simulink model "backstepping"  (R2018a)
settings: Solver=VariableStepAuto  StartTime=0.0  StopTime=500  RelTol=1e-3
values from neighbouring files (symbols this model uses):
  D = 0    [k_func.m]
libraries: simulink_extras x4, sharedutil x3, dspmtrx3 x3
settings Model: Creator=Renz  LastModifiedBy=Renz

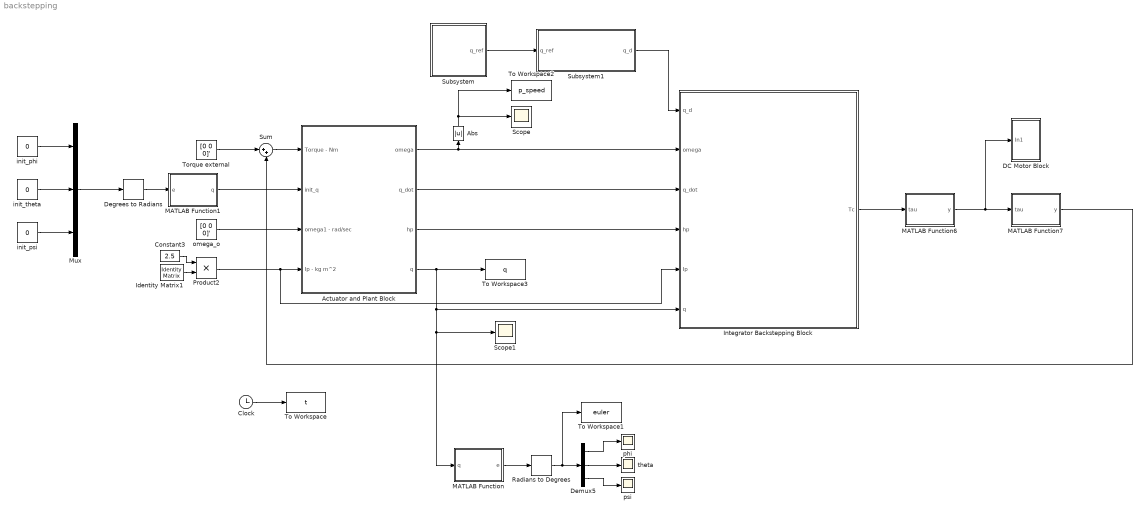
== system backstepping ==
  Abs : Abs
  Actuator and Plant Block : Subsystem
  Clock : Clock
  Constant3 : Constant  Value=2.5
  DC Motor Block : Subsystem
  Degrees to Radians : simulink_extras/Transformations/Degrees to Radians
  Demux5 : Demux  Outputs=3
  Identity Matrix1 : dspmtrx3/Identity Matrix  Inherit=off  N=3  Ts=1  dataType=double  isSigned=on  wordLen=16  udDataType=sfix(16)  fracBitsMode=Best precision  numFracBits=15  OutDataTypeStr=double  LastOutDataTypeStr=double
      settings: SourceProductName=DSP System Toolbox
  Integrator Backstepping Block : Subsystem
  MATLAB Function : MATLAB Function  TreatAsAtomicUnit=on
  MATLAB Function1 : MATLAB Function  TreatAsAtomicUnit=on
  MATLAB Function6 : MATLAB Function  TreatAsAtomicUnit=on
  MATLAB Function7 : MATLAB Function  TreatAsAtomicUnit=on
  Mux : Mux  Inputs=3
  Product2 : Product
  Radians to Degrees : simulink_extras/Transformations/Radians to Degrees
  Scope : Scope
  Scope1 : Scope
  Subsystem : Subsystem
  Subsystem1 : Subsystem
  Sum : Sum  Inputs=|++
  To Workspace : ToWorkspace  VariableName=t  SampleTime=-1
  To Workspace1 : ToWorkspace  VariableName=euler  SampleTime=-1
  To Workspace2 : ToWorkspace  VariableName=p_speed  SampleTime=-1
  To Workspace3 : ToWorkspace  VariableName=q  SampleTime=-1
  Torque external : Constant  Value=[0 0 0]'
  init_phi : Constant  Value=0
  init_psi : Constant  Value=0
  init_theta : Constant  Value=0
  "omega_o " : Constant  Value=[0 0 0]'
  phi : Scope
  psi : Scope
  theta : Scope
  wires:
  Identity Matrix1/1 -> Product2/2
  MATLAB Function1/1(q) -> Actuator and Plant Block/2(init_q)
  init_psi/1 -> Mux/3
  "omega_o "/1 -> Actuator and Plant Block/3(omega1 - rad/sec)
  Sum/1 -> Actuator and Plant Block/1(Torque - Nm)
  init_theta/1 -> Mux/2
  Demux5/3 -> psi/1
  Product2/1 -> Integrator Backstepping Block/5(Ip), Actuator and Plant Block/4(Ip - kg m^2)
  Demux5/1 -> phi/1
  Constant3/1 -> Product2/1
  Clock/1 -> To Workspace/1
  Subsystem/1(q_ref) -> Subsystem1/1(q_ref)
  Actuator and Plant Block/4(q) -> MATLAB Function/1(q), Scope1/1, Integrator Backstepping Block/6(q), To Workspace3/1
  Radians to Degrees/1 -> To Workspace1/1, Demux5/1
  Actuator and Plant Block/1(omega) -> Integrator Backstepping Block/2(omega), Abs/1
  MATLAB Function/1(e) -> Radians to Degrees/1
  Torque external/1 -> Sum/1
  Demux5/2 -> theta/1
  init_phi/1 -> Mux/1
  Degrees to Radians/1 -> MATLAB Function1/1(e)
  Mux/1 -> Degrees to Radians/1
  Abs/1 -> To Workspace2/1, Scope/1
  MATLAB Function7/1(y) -> Sum/2
  MATLAB Function6/1(y) -> MATLAB Function7/1(tau), DC Motor Block/1(In1)
  Subsystem1/1(q_d) -> Integrator Backstepping Block/1(q_d)
  Actuator and Plant Block/2(q_dot) -> Integrator Backstepping Block/3(q_dot)
  Actuator and Plant Block/3(hp) -> Integrator Backstepping Block/4(hp)
  Integrator Backstepping Block/1(Tc) -> MATLAB Function6/1(tau)

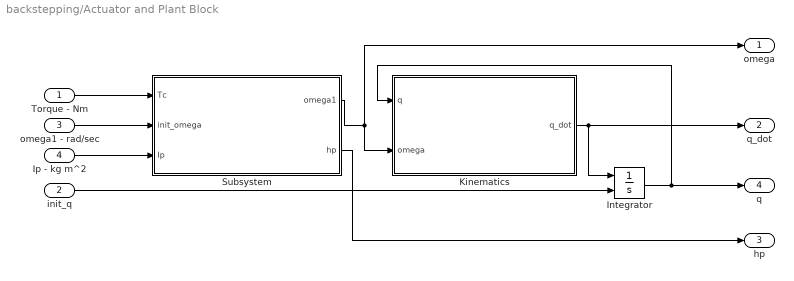
== system backstepping/Actuator and Plant Block ==
  Torque - Nm : Inport
  init_q : Inport  Port=2
  omega1 - rad/sec : Inport  Port=3
  Ip - kg m^2 : Inport  Port=4
  Integrator : Integrator  InitialConditionSource=external
  Kinematics : Subsystem
  Subsystem : Subsystem
  omega : Outport
  q_dot : Outport  Port=2
  hp : Outport  Port=3
  q : Outport  Port=4
  wires:
  Integrator/1 -> Kinematics/1(q), q/1
  Torque - Nm/1 -> Subsystem/1(Tc)
  omega1 - rad/sec/1 -> Subsystem/2(init_omega)
  init_q/1 -> Integrator/2
  Subsystem/1(omega1) -> Kinematics/2(omega), omega/1
  Ip - kg m^2/1 -> Subsystem/3(Ip)
  Kinematics/1(q_dot) -> q_dot/1, Integrator/1
  Subsystem/2(hp) -> hp/1

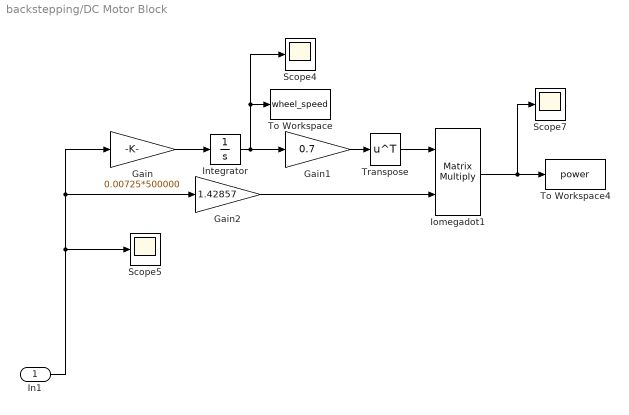
== system backstepping/DC Motor Block ==
  In1 : Inport
  Gain : Gain  Gain=0.00725*500000
  Gain1 : Gain  Gain=0.7
  Gain2 : Gain  Gain=1.42857
  Integrator : Integrator
  Iomegadot1 : Product  Multiplication=Matrix(*)
  Scope4 : Scope
  Scope5 : Scope
  Scope7 : Scope
  To Workspace : ToWorkspace  VariableName=wheel_speed  SampleTime=-1
  To Workspace4 : ToWorkspace  VariableName=power  SampleTime=-1
  Transpose : Math  Operator=transpose  SaturateOnIntegerOverflow=on
  wires:
  Gain/1 -> Integrator/1
  Gain2/1 -> Iomegadot1/2
  Iomegadot1/1 -> Scope7/1, To Workspace4/1
  Transpose/1 -> Iomegadot1/1
  In1/1 -> Scope5/1, Gain2/1, Gain/1
  Integrator/1 -> To Workspace/1, Scope4/1, Gain1/1
  Gain1/1 -> Transpose/1

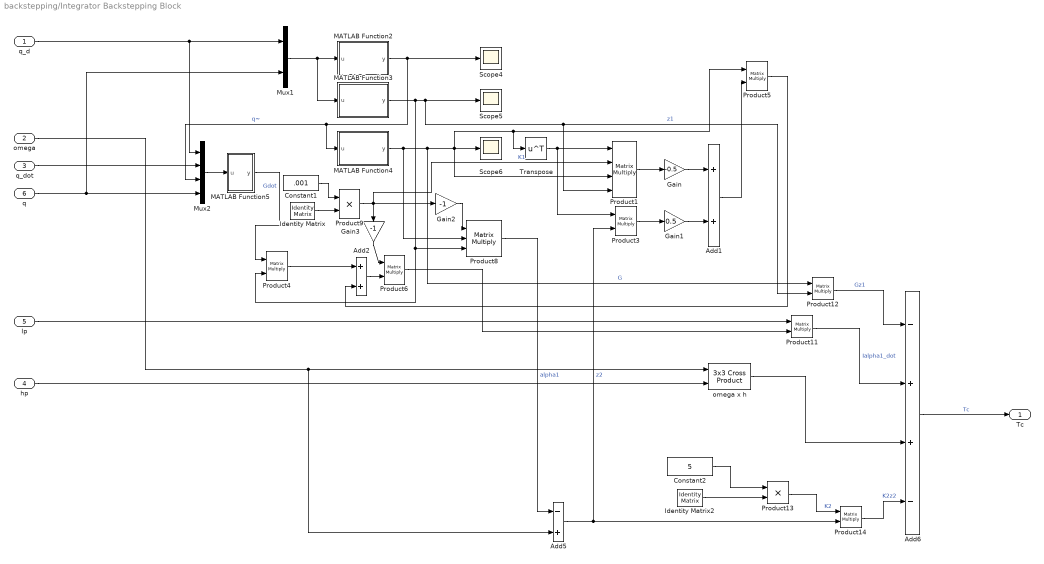
== system backstepping/Integrator Backstepping Block ==
  q_d : Inport
  omega : Inport  Port=2
  q_dot : Inport  Port=3
  hp : Inport  Port=4
  Ip : Inport  Port=5
  q : Inport  Port=6
  Add1 : Sum
  Add2 : Sum
  Add5 : Sum  Inputs=-+
  Add6 : Sum  Inputs=-++-
  Constant1 : Constant  Value=.001
  Constant2 : Constant  Value=5
  Gain : Gain  Gain=-0.5
  Gain1 : Gain  Gain=0.5
  Gain2 : Gain  Gain=-1
  Gain3 : Gain  Gain=-1
  Identity Matrix : dspmtrx3/Identity Matrix  Inherit=off  N=3  Ts=1  dataType=double  isSigned=on  wordLen=16  udDataType=sfix(16)  fracBitsMode=Best precision  numFracBits=15  OutDataTypeStr=double  LastOutDataTypeStr=double
      settings: SourceProductName=DSP System Toolbox
  Identity Matrix2 : dspmtrx3/Identity Matrix  Inherit=off  N=3  Ts=1  dataType=double  isSigned=on  wordLen=16  udDataType=sfix(16)  fracBitsMode=Best precision  numFracBits=15  OutDataTypeStr=double  LastOutDataTypeStr=double
      settings: SourceProductName=DSP System Toolbox
  MATLAB Function2 : MATLAB Function  TreatAsAtomicUnit=on
  MATLAB Function3 : MATLAB Function  TreatAsAtomicUnit=on
  MATLAB Function4 : MATLAB Function  TreatAsAtomicUnit=on
  MATLAB Function5 : MATLAB Function  TreatAsAtomicUnit=on
  Mux1 : Mux  Inputs=2
  Mux2 : Mux
  Product1 : Product  Inputs=4  Multiplication=Matrix(*)
  Product{3..6,11..12,14} (7 alike) : Product  Multiplication=Matrix(*)
  Product13 : Product
  Product8 : Product  Inputs=3  Multiplication=Matrix(*)
  Product9 : Product
  Scope4 : Scope
  Scope5 : Scope
  Scope6 : Scope
  Transpose : Math  Operator=transpose  SaturateOnIntegerOverflow=on
  omega x h : sharedutil/3x3 Cross Product  aMode=aMode
      settings: SourceProductBaseCode=AE
  Tc : Outport
  wires:
  Ip/1 -> Product11/1
  Constant2/1 -> Product13/1
  MATLAB Function3/1(y) -> Product4/2, Product8/3, Product1/4, Product12/2, Scope5/1  "z1"
  MATLAB Function4/1(y) -> Product8/2, Product12/1, Product1/3, Product5/1, Transpose/1, Scope6/1  "G"
  Add5/1 -> Product3/2, Product14/2  "z2"
  Product11/1 -> Add6/2  "Ialpha1_dot"
  MATLAB Function5/1(y) -> Product4/1  "Gdot"
  q_d/1 -> Mux2/1, Mux1/1
  MATLAB Function2/1(y) -> MATLAB Function4/1(u), Mux2/3, Scope4/1  "q~"
  Product12/1 -> Add6/1  "Gz1"
  Gain3/1 -> Product6/1
  Add1/1 -> Product5/2
  Gain1/1 -> Add1/2
  Identity Matrix/1 -> Product9/2
  Transpose/1 -> Product3/1, Product1/1
  Mux1/1 -> MATLAB Function3/1(u), MATLAB Function2/1(u)
  Product9/1 -> Product1/2, Gain3/1, Gain2/1  "K1"
  Identity Matrix2/1 -> Product13/2
  Product13/1 -> Product14/1  "K2"
  Gain/1 -> Add1/1
  q/1 -> Mux1/2, Mux2/4
  Product8/1 -> Add5/1  "alpha1"
  Product3/1 -> Gain1/1
  hp/1 -> omega x h/2
  Product6/1 -> Product11/2
  q_dot/1 -> Mux2/2
  Mux2/1 -> MATLAB Function5/1(u)
  Product5/1 -> Add2/2
  omega/1 -> omega x h/1, Add5/2
  Product1/1 -> Gain/1
  Product14/1 -> Add6/4  "K2z2"
  Gain2/1 -> Product8/1
  omega x h/1 -> Add6/3
  Constant1/1 -> Product9/1
  Add2/1 -> Product6/2
  Product4/1 -> Add2/1
  Add6/1 -> Tc/1  "Tc"

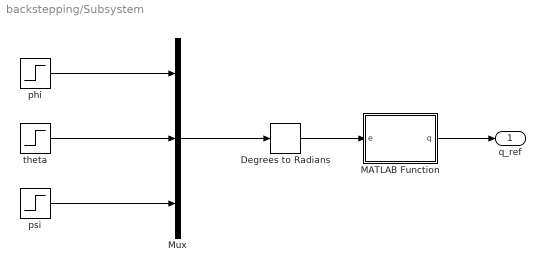
== system backstepping/Subsystem ==
  Degrees to Radians : simulink_extras/Transformations/Degrees to Radians
  MATLAB Function : MATLAB Function  TreatAsAtomicUnit=on
  Mux : Mux  Inputs=3
  phi : Step  Before=80  After=80  SampleTime=0
  psi : Step  Before=60  After=60  SampleTime=0
  theta : Step  Before=40  After=40  SampleTime=0
  q_ref : Outport
  wires:
  Mux/1 -> Degrees to Radians/1
  psi/1 -> Mux/3
  phi/1 -> Mux/1
  theta/1 -> Mux/2
  MATLAB Function/1(q) -> q_ref/1
  Degrees to Radians/1 -> MATLAB Function/1(e)

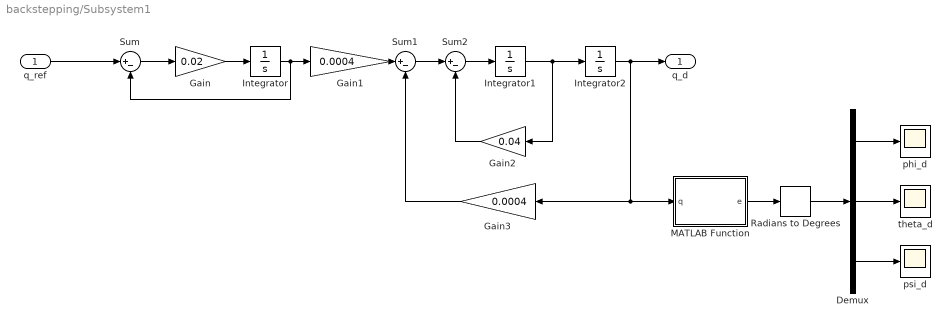
== system backstepping/Subsystem1 ==
  q_ref : Inport
  Demux : Demux  Outputs=3
  Gain : Gain  Gain=0.02
  Gain1 : Gain  Gain=0.0004
  Gain2 : Gain  Gain=0.04
  Gain3 : Gain  Gain=0.0004
  Integrator : Integrator
  Integrator1 : Integrator
  Integrator2 : Integrator
  MATLAB Function : MATLAB Function  TreatAsAtomicUnit=on
  Radians to Degrees : simulink_extras/Transformations/Radians to Degrees
  Sum : Sum  Inputs=|+-
  Sum1 : Sum  Inputs=|+-
  Sum2 : Sum  Inputs=|+-
  phi_d : Scope
  psi_d : Scope
  theta_d : Scope
  q_d : Outport
  wires:
  Demux/3 -> psi_d/1
  Gain1/1 -> Sum1/1
  Sum/1 -> Gain/1
  Gain2/1 -> Sum2/2
  Demux/2 -> theta_d/1
  Gain/1 -> Integrator/1
  Integrator/1 -> Gain1/1, Sum/2
  Sum1/1 -> Sum2/1
  Gain3/1 -> Sum1/2
  Integrator1/1 -> Gain2/1, Integrator2/1
  Sum2/1 -> Integrator1/1
  q_ref/1 -> Sum/1
  Demux/1 -> phi_d/1
  Radians to Degrees/1 -> Demux/1
  Integrator2/1 -> q_d/1, MATLAB Function/1(q), Gain3/1
  MATLAB Function/1(e) -> Radians to Degrees/1

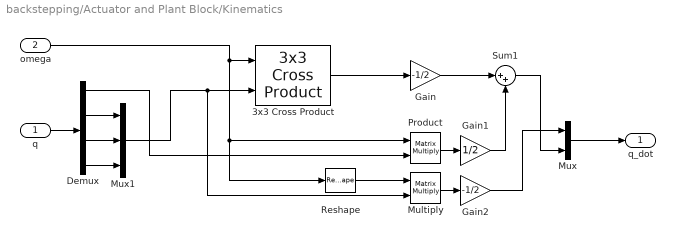
== system backstepping/Actuator and Plant Block/Kinematics ==
  q : Inport
  omega : Inport  Port=2
  3x3 Cross Product : sharedutil/3x3 Cross Product  aMode=aMode
      settings: SourceProductBaseCode=AE
  Demux : Demux
  Gain : Gain  Gain=-1/2
  Gain1 : Gain  Gain=1/2
  Gain2 : Gain  Gain=-1/2
  Multiply : Product  Multiplication=Matrix(*)
  Mux : Mux  Inputs=2
  Mux1 : Mux  Inputs=3
  Product : Product  Multiplication=Matrix(*)
  Reshape : Reshape  OutputDimensionality=Row vector (2-D)
  Sum1 : Sum  Inputs=|++
  q_dot : Outport
  wires:
  omega/1 -> 3x3 Cross Product/1, Product/1, Reshape/1
  q/1 -> Demux/1
  Mux1/1 -> Multiply/2, 3x3 Cross Product/2
  Gain1/1 -> Sum1/2
  3x3 Cross Product/1 -> Gain/1
  Product/1 -> Gain1/1
  Multiply/1 -> Gain2/1
  Gain/1 -> Sum1/1
  Demux/1 -> Product/2
  Reshape/1 -> Multiply/1
  Mux/1 -> q_dot/1
  Sum1/1 -> Mux/2
  Gain2/1 -> Mux/1
  Demux/2 -> Mux1/1
  Demux/3 -> Mux1/2
  Demux/4 -> Mux1/3

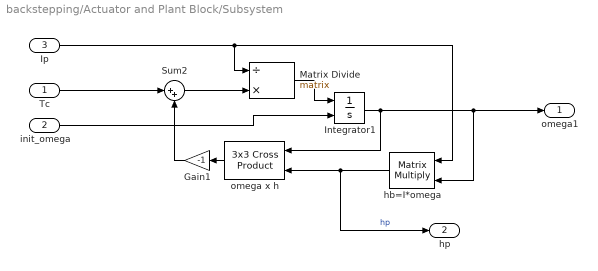
== system backstepping/Actuator and Plant Block/Subsystem ==
  Tc : Inport
  init_omega : Inport  Port=2
  Ip : Inport  Port=3
  Gain1 : Gain  Gain=-1
  Integrator1 : Integrator  InitialConditionSource=external  ZeroCross=off
  Matrix Divide : Product  Inputs=/*  Multiplication=Matrix(*)
  Sum2 : Sum  Inputs=|++
  hb=I*omega : Product  Multiplication=Matrix(*)
  omega x h : sharedutil/3x3 Cross Product  aMode=aMode
      settings: SourceProductBaseCode=AE
  omega1 : Outport
  hp : Outport  Port=2
  wires:
  Gain1/1 -> Sum2/2
  Integrator1/1 -> omega x h/1, omega1/1, hb=I*omega/2
  init_omega/1 -> Integrator1/2
  Sum2/1 -> Matrix Divide/2
  hb=I*omega/1 -> hp/1, omega x h/2  "hp"
  omega x h/1 -> Gain1/1
  Tc/1 -> Sum2/1
  Matrix Divide/1 -> Integrator1/1
  Ip/1 -> Matrix Divide/1, hb=I*omega/1

== matlab function backstepping/Subsystem1/MATLAB Function ==
  data: q input; e output
function e = quat2euler(q)

q0 = q(1,:);
q1 = q(2,:);
q2 = q(3,:);
q3 = q(4,:);

phi = atan((2*(q2*q3 + q0*q1))/(q0^2 - q1^2 - q2^2 + q3^2)); 
theta = asin(-2*(q1*q3 - q0*q2));
psi = atan((2*(q1*q2 + q0*q3))/(q0^2 + q1^2 -q2^2 - q3^2)); 

e = [phi;theta;psi];

end

== matlab function backstepping/Subsystem/MATLAB Function ==
  data: e input; q output
function q = euler2quat(e)

e1 = 0.5*e(1,:);
e2 = 0.5*e(2,:);
e3 = 0.5*e(3,:);

q0 = (sin(e1)*sin(e2)*sin(e3)) + (cos(e1)*cos(e2)*cos(e3));
q1 = (-sin(e2)*sin(e3)*cos(e1)) + (sin(e1)*cos(e2)*cos(e3));
q2 = (sin(e1)*cos(e2)*sin(e3)) + (sin(e2)*cos(e1)*cos(e3));
q3 = (sin(e3)*cos(e1)*cos(e2)) - (sin(e1)*sin(e2)*cos(e3));

q = [q0;q1;q2;q3];

end

== matlab function backstepping/MATLAB Function1 ==
  data: e input; q output
function q = euler2quat(e)

e1 = 0.5*e(1,:);
e2 = 0.5*e(2,:);
e3 = 0.5*e(3,:);

q0 = (sin(e1)*sin(e2)*sin(e3)) + (cos(e1)*cos(e2)*cos(e3));
q1 = (-sin(e2)*sin(e3)*cos(e1)) + (sin(e1)*cos(e2)*cos(e3));
q2 = (sin(e1)*cos(e2)*sin(e3)) + (sin(e2)*cos(e1)*cos(e3));
q3 = (sin(e3)*cos(e1)*cos(e2)) - (sin(e1)*sin(e2)*cos(e3));

q = [q0;q1;q2;q3];

end

== matlab function backstepping/Integrator Backstepping Block/MATLAB Function2 ==
  data: u input; y output
function y = q_func(u)
%d - desired quaternions, a - actual quaternions
d1 = u(1,:);
d2 = u(2,:);
d3 = u(3,:);
d4 = u(4,:);
a1 = u(5,:);
a2 = u(6,:);
a3 = u(7,:);
a4 = u(8,:);
epsi_d = [d2;d3;d4];
epsi_a = [a2;a3;a4];
S = cross(epsi_d);
up = (a1*d1) + (epsi_d'*epsi_a);
down = (d1*epsi_a) - (a1*epsi_d) - (S*epsi_a);
y = [up;down];

== matlab function backstepping/Integrator Backstepping Block/MATLAB Function3 ==
  data: u input; y output
function y = z1_func(u)
%d - desired quaternions, a - actual quaternions
d1 = u(1,:);
d2 = u(2,:);
d3 = u(3,:);
d4 = u(4,:);
a1 = u(5,:);
a2 = u(6,:);
a3 = u(7,:);
a4 = u(8,:);
epsi_d = [d2;d3;d4];
epsi_a = [a2;a3;a4];
S = cross(epsi_d);
up = (a1*d1) + (epsi_d'*epsi_a);
down = (d1*epsi_a) - (a1*epsi_d) - (S*epsi_a);
y = [1-abs(up);down];

== matlab function backstepping/MATLAB Function ==
  data: q input; e output
function e = quat2euler(q)

q0 = q(1,:);
q1 = q(2,:);
q2 = q(3,:);
q3 = q(4,:);

phi = atan((2*(q2*q3 + q0*q1))/(q0^2 - q1^2 - q2^2 + q3^2)); 
theta = asin(-2*(q1*q3 - q0*q2));
psi = atan((2*(q1*q2 + q0*q3))/(q0^2 + q1^2 -q2^2 - q3^2)); 

e = [phi;theta;psi];

end

== matlab function backstepping/Integrator Backstepping Block/MATLAB Function4 ==
  data: u input; y output
function y = G_func(u)
%d - q~
I = 2.5*eye(3);
d1 = u(1,:);
d2 = u(2,:);
d3 = u(3,:);
d4 = u(4,:);
epsi = [d2;d3;d4];
S = cross(epsi);
up = signum(d1)*epsi;
down = (d1*I) + S;
y = [up';down]';

== matlab function backstepping/Integrator Backstepping Block/MATLAB Function5 ==
  data: u input; y output
function y = qdot_func(u)
%d - desired quaternions, a - actual quaternions dot
I = 2.5*eye(3);
d1 = u(1,:);
d2 = u(2,:);
d3 = u(3,:);
d4 = u(4,:);
a1 = u(5,:);
a2 = u(6,:);
a3 = u(7,:);
a4 = u(8,:);
n = u(9,:);
n_act = u(13,:);
epsi_d = [d2;d3;d4];
epsi_a = [a2;a3;a4];
S_d = cross(epsi_d);
S_a = cross(epsi_a);

eta_up = -signum(n)*epsi_d'*a1;
eta_down = (d1*I - S_d)*a1;
eta = [eta_up; eta_down]';
epsi_up = signum(n)*(d1*epsi_a' -epsi_d'*(n_act*I +S_a));
epsi_down = (d1*I - S_d)*S_a + epsi_d*epsi_a';
epsi = [epsi_up; epsi_down]';
y = eta + epsi;

== matlab function backstepping/MATLAB Function6 ==
  data: tau input; y output
function y = control_alloc(tau)
K =[1 0 0 0 
    0 1 0 0 
    0 0 1 0 
    0 0 0 1];
T = [0.57735, -0.57735, -0.57735, 0.57735; 0.57735, -0.57735, 0.57735, -0.57735; 0.57735, 0.57735, -0.57735, -0.57735];
W = [1 0 0 0     
    0 1 0 0      
    0 0 1 0      
    0 0 0 1];


y = ucalloc(K,T,W,tau);

== matlab function backstepping/MATLAB Function7 ==
  data: tau input; y output
function y = torque(tau)
L = [0.57735, -0.57735, -0.57735, 0.57735; 0.57735, -0.57735, 0.57735, -0.57735; 0.57735, 0.57735, -0.57735, -0.57735];


y = L*tau;
